simulink model "mIkinValidator"  (R2021a)
settings: Solver=VariableStepAuto  StartTime=0.0  StopTime=inf  RelTol=1e-3
undefined symbols (not defined in the file): adA, adAlpha, adD, adHome6rad, adLinkLenghts, adMotorLimits, adOffset, adPoints, adWeight, adWS, Levenberg, Marquardt
libraries: robotcorelib x3, robotmaniplib x2, simulink x1
settings Model: Creator=angelo  LastModifiedBy=angelo

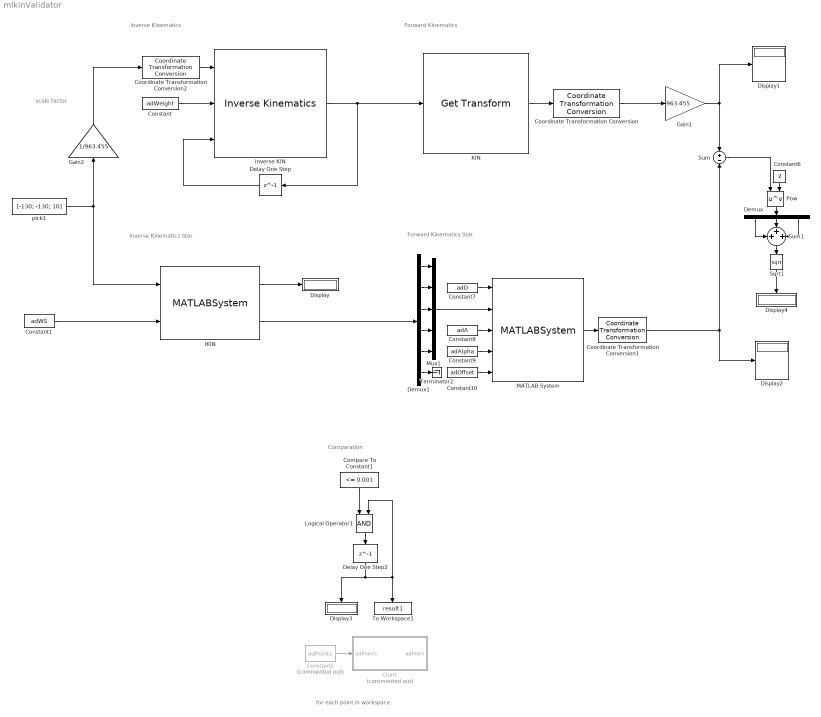
== system mIkinValidator ==
  note: for each point in workspace
  note: scale factor
  note: Inverse Kinematics
  note: Forward Kinematics Star
  note: Forward Kinematics
  note: Inverse Kinematics Star
  note: Comparation
  Chart : Stateflow chart  Commented=on  TreatAsAtomicUnit=on
  Compare To Constant1 : simulink/Logic and Bit Operations/Compare To Constant  relop=<=  const=0.001  OutDataTypeStr=boolean
  Constant : Constant  Value=adWeight
  Constant1 : Constant  Value=adWS
  Constant10 : Constant  Value=adOffset
  Constant2 : Constant  Commented=on  Value=adPoints
  Constant6 : Constant  Value=2
  Constant7 : Constant  Value=adD
  Constant8 : Constant  Value=adA
  Constant9 : Constant  Value=adAlpha
  Coordinate Transformation Conversion : robotcorelib/Coordinate Transformation Conversion  InputRepresentation=Homogeneous Transformation  InputEulerSequence=ZYX  ShowTrVecInputPort=on  OutputRepresentation=Translation Vector  OutputEulerSequence=ZYX  ShowTrVecOutputPort=on  SimulateUsing=Interpreted execution
      settings: SourceProductBaseCode=NV,RO,RR,UV
  Coordinate Transformation Conversion1 : robotcorelib/Coordinate Transformation Conversion  InputRepresentation=Homogeneous Transformation  InputEulerSequence=ZYX  ShowTrVecInputPort=on  OutputRepresentation=Translation Vector  OutputEulerSequence=ZYX  ShowTrVecOutputPort=on  SimulateUsing=Interpreted execution
      settings: SourceProductBaseCode=NV,RO,RR,UV
  Coordinate Transformation Conversion2 : robotcorelib/Coordinate Transformation Conversion  InputRepresentation=Translation Vector  InputEulerSequence=ZYX  ShowTrVecInputPort=on  OutputRepresentation=Homogeneous Transformation  OutputEulerSequence=ZYX  ShowTrVecOutputPort=on  SimulateUsing=Interpreted execution
      settings: SourceProductBaseCode=NV,RO,RR,UV
  Delay One Step : Delay  DelayLength=1  InitialCondition=adHome6rad
  Delay One Step2 : Delay  DelayLength=1  InitialCondition=true
  Demux : Demux  Outputs=3
  Demux1 : Demux  Outputs=6
  Display{,1..4} (5 alike) : Display
  Gain1 : Gain  Gain=963.455
  Gain2 : Gain  Gain=1/963.455
  IKIN : MATLABSystem  System=oIKINSolver  adHomeDeg=adHome6deg  nGroundLength=adLinkLenghts(1)  nArmLength=adLinkLenghts(2)  nForearmLength=adLinkLenghts(3)  nHandLength=adLinkLenghts(4)  adBaseMinMaxDeg=adMotorLimits(1,:)  adShoulderMinMaxDeg=adMotorLimits(2,:)  adElbowMinMaxDeg=adMotorLimits(3,:)  adPitchMinMaxDeg=adMotorLimits(4,:)  adRollMinMaxDeg=adMotorLimits(5,:)  SimulateUsing=Code generation
      mask Type: oIKINSolver
      mask Display:
      | disp('oIKINSolver');
      | port_label('input',1,'adPoint');
      | port_label('input',2,'adWS');
      | port_label('output',1,'bFlag');
      | port_label('output',2,'adJC');
  Inverse KIN : robotmaniplib/Inverse Kinematics  RigidBodyTree=oBraccio6dofee  EndEffector=ee  ShowInfo=off  SolverName=Levenberg-Marquardt  EnforceJointLimits=on  MaxIterations=1500  MaxTime=10  GradientTolerance=1e-7  SolutionTolerance=1e-6  StepTolerance=1e-14  ErrorChangeTolerance=1e-12  UseErrorDamping=on  DampingBias=0.0025  SimulateUsing=Interpreted execution
  KIN : robotmaniplib/Get Transform  RigidBodyTree=oBraccio6dofee  SourceBody=ee  TargetBody=base_link  SimulateUsing=Interpreted execution
  Logical Operator1 : Logic  AllPortsSameDT=off  OutDataTypeStr=boolean
  MATLAB System : MATLABSystem  System=oKINSolver  adHomeDeg=adHome6deg  nGroundLength=adLinkLenghts(1)  nArmLength=adLinkLenghts(2)  nForearmLength=adLinkLenghts(3)  nHandLength=adLinkLenghts(4)  adBaseMinMaxDeg=adMotorLimits(1,:)  adShoulderMinMaxDeg=adMotorLimits(2,:)  adElbowMinMaxDeg=adMotorLimits(3,:)  adPitchMinMaxDeg=adMotorLimits(4,:)  adRollMinMaxDeg=adMotorLimits(5,:)  SimulateUsing=Code generation
      mask Type: oKINSolver
      mask Display:
      | disp('oKINSolver');
      | port_label('input',1,'adD');
      | port_label('input',2,'adQ');
      | port_label('input',3,'adA');
      | port_label('input',4,'adAlpha');
      | port_label('input',5,'adOffset');
      | port_label('output',1,'adT');
  Mux1 : Mux  Inputs=5
  Pow : Math  Operator=pow  RndMeth=Zero  SaturateOnIntegerOverflow=on
  Sqrt1 : Sqrt  SaturateOnIntegerOverflow=on
  Sum : Sum  Inputs=+|-
  Sum1 : Sum  Inputs=+++
  Terminator2 : Terminator
  To Workspace1 : ToWorkspace  VariableName=result1  SaveFormat=Timeseries  SampleTime=-1
  pick1 : Constant  Value=[-130; -130; 10]
  wires:
  Constant/1 -> Inverse KIN/2
  Delay One Step/1 -> Inverse KIN/3
  Inverse KIN/1 -> Delay One Step/1, KIN/1
  Coordinate Transformation Conversion2/1 -> Inverse KIN/1
  IKIN/2 -> Demux1/1
  Constant1/1 -> IKIN/2
  IKIN/1 -> Display/1
  KIN/1 -> Coordinate Transformation Conversion/1
  Demux1/6 -> Terminator2/1
  Demux1/5 -> Mux1/5
  Demux1/2 -> Mux1/2
  Mux1/1 -> MATLAB System/2
  Demux1/3 -> Mux1/3
  Demux1/1 -> Mux1/1
  Demux1/4 -> Mux1/4
  Coordinate Transformation Conversion/1 -> Gain1/1
  Gain2/1 -> Coordinate Transformation Conversion2/1
  Coordinate Transformation Conversion1/1 -> Display2/1, Sum/2
  Demux/2 -> Sum1/2
  Demux/1 -> Sum1/1
  Demux/3 -> Sum1/3
  Sum/1 -> Pow/1
  Pow/1 -> Demux/1
  Sum1/1 -> Sqrt1/1
  Constant6/1 -> Pow/2
  Constant10/1 -> MATLAB System/5
  Constant8/1 -> MATLAB System/3
  Constant9/1 -> MATLAB System/4
  Constant7/1 -> MATLAB System/1
  MATLAB System/1 -> Coordinate Transformation Conversion1/1
  Constant2/1 -> Chart/1(adPoints)
  pick1/1 -> IKIN/1, Gain2/1
  Gain1/1 -> Display1/1, Sum/1
  Logical Operator1/1 -> Delay One Step2/1
  Compare To Constant1/1 -> Logical Operator1/1
  Delay One Step2/1 -> Display3/1, To Workspace1/1, Logical Operator1/2
  ? -> Compare To Constant1/1
  Sqrt1/1 -> Display4/1

== stateflow chart mIkinValidator/Chart ==
  data: adPoints input; adPoint output
